simulink model "Model_AC_TES_Double_Coil"  (R2025b)
settings: Solver=VariableStepAuto  StartTime=0.0  StopTime=3600*9  RelTol=1e-3
model workspace (MAT data in the model file):
  COP = 3.9
  Delayfan = [30 1]
  P1 = 1.05
  P2 = 1.91
  P3 = 1.91
  P4 = 1.05
  Q_Cond = 4.361
  Q_Evap = 3.471
  T1 = 12
  T2 = 37.72
  T3 = 29.61
  T4 = 7.9
  T_Enviroment_C = 27.5
  T_Room_int_C = 28.6
  T_Tank_int_c = 30
  Wall_h_in = 12
  Wall_h_out = 38
  h1 = 522.3
  h2 = 528.6
  h3 = 253.4
  h4 = 253.4
  m_dot = 0.014
libraries: fl_lib x102, nesl_utility x62, SimscapeFluids_lib x31
(part 2 of 3)

== system Model_AC_TES_Double_Coil/22-12-2025 ==
  Clock2 : Clock
  Clock3 : Clock
  Constant1 : Constant
  Constant2 : Constant  Value=0
  Constant3 : Constant  Value=0
  Switch2 : Switch  Criteria=u2 > Threshold  Threshold=3600*10  SaturateOnIntegerOverflow=off  InputSameDT=off
  Switch3 : Switch  Criteria=u2 > Threshold  Threshold=3600*17  SaturateOnIntegerOverflow=off  InputSameDT=off
  Out1 : Outport
  wires:
  Constant3/1 -> Switch2/3
  Constant1/1 -> Switch2/1
  Clock2/1 -> Switch2/2
  Switch3/1 -> Out1/1
  Constant2/1 -> Switch3/1
  Clock3/1 -> Switch3/2
  Switch2/1 -> Switch3/3

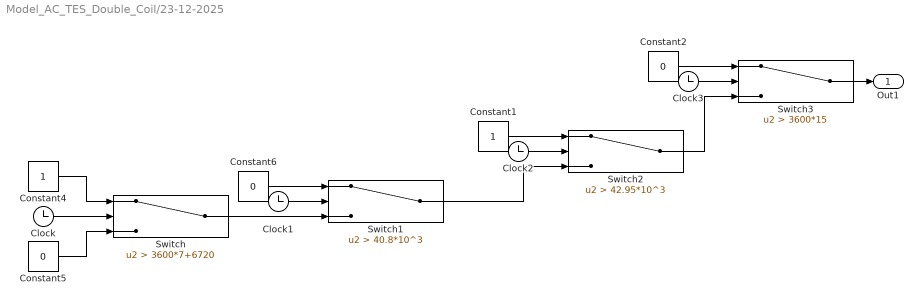
== system Model_AC_TES_Double_Coil/23-12-2025 ==
  Clock{,1..3} (4 alike) : Clock
  Constant1 : Constant
  Constant2 : Constant  Value=0
  Constant4 : Constant
  Constant5 : Constant  Value=0
  Constant6 : Constant  Value=0
  Switch : Switch  Criteria=u2 > Threshold  Threshold=3600*7+6720  SaturateOnIntegerOverflow=off  InputSameDT=off
  Switch1 : Switch  Criteria=u2 > Threshold  Threshold=40.8*10^3  SaturateOnIntegerOverflow=off  InputSameDT=off
  Switch2 : Switch  Criteria=u2 > Threshold  Threshold=42.95*10^3  SaturateOnIntegerOverflow=off  InputSameDT=off
  Switch3 : Switch  Criteria=u2 > Threshold  Threshold=3600*15  SaturateOnIntegerOverflow=off  InputSameDT=off
  Out1 : Outport
  wires:
  Constant6/1 -> Switch1/1
  Clock1/1 -> Switch1/2
  Switch/1 -> Switch1/3
  Constant4/1 -> Switch/1
  Clock/1 -> Switch/2
  Switch1/1 -> Switch2/3
  Constant5/1 -> Switch/3
  Constant1/1 -> Switch2/1
  Clock2/1 -> Switch2/2
  Switch3/1 -> Out1/1
  Constant2/1 -> Switch3/1
  Clock3/1 -> Switch3/2
  Switch2/1 -> Switch3/3

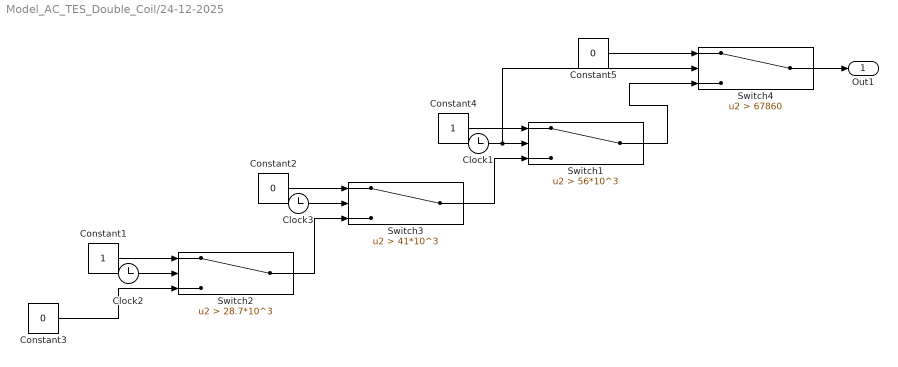
== system Model_AC_TES_Double_Coil/24-12-2025 ==
  Clock1 : Clock
  Clock2 : Clock
  Clock3 : Clock
  Constant1 : Constant
  Constant2 : Constant  Value=0
  Constant3 : Constant  Value=0
  Constant4 : Constant
  Constant5 : Constant  Value=0
  Switch1 : Switch  Criteria=u2 > Threshold  Threshold=56*10^3  SaturateOnIntegerOverflow=off  InputSameDT=off
  Switch2 : Switch  Criteria=u2 > Threshold  Threshold=28.7*10^3  SaturateOnIntegerOverflow=off  InputSameDT=off
  Switch3 : Switch  Criteria=u2 > Threshold  Threshold=41*10^3  SaturateOnIntegerOverflow=off  InputSameDT=off
  Switch4 : Switch  Criteria=u2 > Threshold  Threshold=67860  SaturateOnIntegerOverflow=off  InputSameDT=off
  Out1 : Outport
  wires:
  Constant3/1 -> Switch2/3
  Constant1/1 -> Switch2/1
  Clock2/1 -> Switch2/2
  Constant2/1 -> Switch3/1
  Clock3/1 -> Switch3/2
  Switch2/1 -> Switch3/3
  Switch1/1 -> Switch4/3
  Constant4/1 -> Switch1/1
  Clock1/1 -> Switch4/2, Switch1/2
  Switch3/1 -> Switch1/3
  Constant5/1 -> Switch4/1
  Switch4/1 -> Out1/1

== system Model_AC_TES_Double_Coil/25-12-2025 ==
  Clock1 : Clock
  Constant1 : Constant  Value=0
  Constant4 : Constant
  Constant5 : Constant  Value=0
  Switch1 : Switch  Criteria=u2 > Threshold  Threshold=28500  SaturateOnIntegerOverflow=off  InputSameDT=off
  Switch4 : Switch  Criteria=u2 > Threshold  Threshold=41600  SaturateOnIntegerOverflow=off  InputSameDT=off
  Out1 : Outport
  wires:
  Switch1/1 -> Switch4/3
  Constant4/1 -> Switch1/1
  Clock1/1 -> Switch4/2, Switch1/2
  Constant1/1 -> Switch1/3
  Constant5/1 -> Switch4/1
  Switch4/1 -> Out1/1

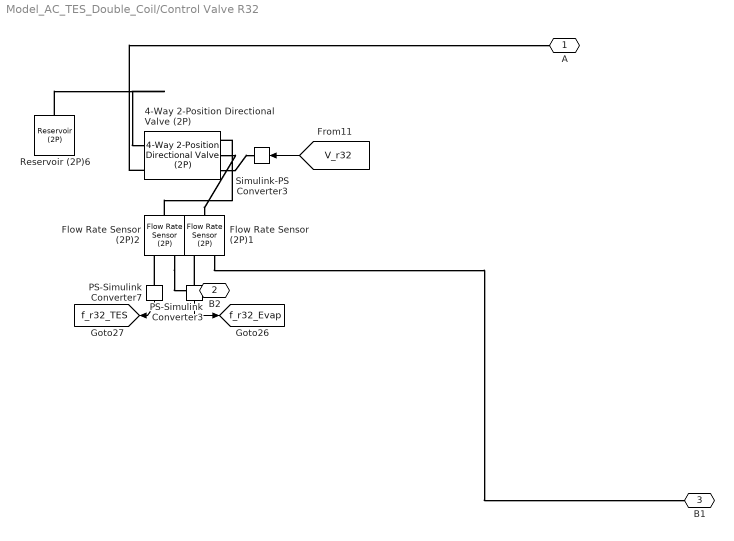
== system Model_AC_TES_Double_Coil/Control Valve R32 ==
  4-Way 2-Position Directional Valve (2P) : SimscapeFluids_lib/Two-Phase Fluid/Valves & Orifices/Directional Control Valves/4-Way 2-Position Directional Valve (2P)  open_orifices_pos=fluids.two_phase_fluid.valves_orifices.directional_control_valves.enum.OpenOrifices4Way2Position.PA  open_orifices_neg=fluids.two_phase_fluid.valves_orifices.directional_control_valves.enum.OpenOrifices4Way2Position.PB  area_spec=fluids.two_phase_fluid.valves_orifices.directional_control_valves.enum.AreaSpec.Identical  liquid_valve_parameterization=fluids.two_phase_fluid.valves_orifices.directional_control_valves.enum.LiquidOrificeParameterization.LinearArea  del_S_max=0.005 m  mdot_nominal_max=0.1 kg/s  delta_p_nominal_max=0.001 MPa  energy_spec=foundation.enum.energy_spec.temperature  p_inlet=0.101325 MPa  T_inlet=293.15 K  x_inlet=0  alpha_inlet=0  h_inlet=400 kJ/kg  u_inlet=400 kJ/kg  valve_area_max=1e-4 m^2  del_S_TLU=[0, .00125, .0025, .00375, .005] m  valve_area_TLU=[1e-10, 1e-05, 4e-05, 6e-05, .0001] m^2  Cd=0.64  pressure_recovery=false  leakage_fraction=1e-6  smoothing_factor=0.01  B_lam=0.999  tau_x=0.1 s  area=0.01 m^2  S_max_PA=0.01 m  del_S_max_PA=0.005 m  mdot_nominal_max_PA=0.1 kg/s  delta_p_nominal_max_PA=0.001 MPa  energy_spec_PA=foundation.enum.energy_spec.temperature  p_inlet_PA=0.101325 MPa  T_inlet_PA=293.15 K  x_inlet_PA=0  alpha_inlet_PA=0  h_inlet_PA=400 kJ/kg  u_inlet_PA=400 kJ/kg  valve_area_max_PA=1e-4 m^2  del_S_TLU_PA=[0, .00125, .0025, .00375, .005] m  valve_area_TLU_PA=[1e-10, 1e-05, 4e-05, 6e-05, .0001] m^2  mdot_nominal_const_PA=0.1 kg/s  delta_p_nominal_const_PA=0.001 MPa  valve_area_const_PA=1e-4 m^2  S_max_PB=0.01 m  del_S_max_PB=0.005 m  mdot_nominal_max_PB=0.1 kg/s  delta_p_nominal_max_PB=0.001 MPa  energy_spec_PB=foundation.enum.energy_spec.temperature  p_inlet_PB=0.101325 MPa  T_inlet_PB=293.15 K  x_inlet_PB=0  alpha_inlet_PB=0  h_inlet_PB=400 kJ/kg  u_inlet_PB=400 kJ/kg  valve_area_max_PB=1e-4 m^2  del_S_TLU_PB=[0, .00125, .0025, .00375, .005] m  valve_area_TLU_PB=[1e-10, 1e-05, 4e-05, 6e-05, .0001] m^2  mdot_nominal_const_PB=0.1 kg/s  delta_p_nominal_const_PB=0.001 MPa  valve_area_const_PB=1e-4 m^2  S_max_AT=-5e-3 m  del_S_max_AT=0.005 m  mdot_nominal_max_AT=0.1 kg/s  delta_p_nominal_max_AT=0.001 MPa  energy_spec_AT=foundation.enum.energy_spec.temperature  p_inlet_AT=0.101325 MPa  T_inlet_AT=293.15 K  x_inlet_AT=0  alpha_inlet_AT=0  h_inlet_AT=400 kJ/kg  u_inlet_AT=400 kJ/kg  valve_area_max_AT=1e-4 m^2  del_S_TLU_AT=[0, .00125, .0025, .00375, .005] m  valve_area_TLU_AT=[1e-10, 1e-05, 4e-05, 6e-05, .0001] m^2  mdot_nominal_const_AT=0.1 kg/s  delta_p_nominal_const_AT=0.001 MPa  valve_area_const_AT=1e-4 m^2  S_max_BT=5e-3 m  del_S_max_BT=0.005 m  mdot_nominal_max_BT=0.1 kg/s  delta_p_nominal_max_BT=0.001 MPa  energy_spec_BT=foundation.enum.energy_spec.temperature  p_inlet_BT=0.101325 MPa  T_inlet_BT=293.15 K  x_inlet_BT=0  alpha_inlet_BT=0  h_inlet_BT=400 kJ/kg  u_inlet_BT=400 kJ/kg  valve_area_max_BT=1e-4 m^2  del_S_TLU_BT=[0, .00125, .0025, .00375, .005] m  valve_area_TLU_BT=[1e-10, 1e-05, 4e-05, 6e-05, .0001] m^2  mdot_nominal_const_BT=0.1 kg/s  delta_p_nominal_const_BT=0.001 MPa  valve_area_const_BT=1e-4 m^2  vapor_valve_parameterization=fluids.two_phase_fluid.valves_orifices.enum.VaporOrificeParameterization.Cv  opening_characteristic=fluids.two_phase_fluid.valves_orifices.enum.OpeningCharacteristics.Linear  Cv_max=4  del_S_Cv_TLU=[0, .001, .002, .003, .004, .005] m  Cv_TLU=[1e-06, .8, 1.6, 2.4, 3.2, 4]  xT_Cv=0.7  Kv_max=3.6  del_S_Kv_TLU=[0, .001, .002, .003, .004, .005] m  Kv_TLU=[1e-06, .72, 1.44, 2.16, 2.88, 3.6]  xT_Kv=0.7  orifice_area_max=1e-4 m^2  del_S_orifice_area_TLU=[0, .001, .002, .003, .004, .005] m  orifice_area_TLU=[1e-10, 2e-05, 4e-05, 6e-05, 8e-05, .0001] m^2  Cv_const_PA=4  Cv_max_PA=4  del_S_Cv_TLU_PA=[0, .001, .002, .003, .004, .005] m  Cv_TLU_PA=[1e-06, .8, 1.6, 2.4, 3.2, 4]  xT_Cv_PA=0.7  Kv_const_PA=3.6  Kv_max_PA=3.6  del_S_Kv_TLU_PA=[0, .001, .002, .003, .004, .005] m  Kv_TLU_PA=[1e-06, .72, 1.44, 2.16, 2.88, 3.6]  xT_Kv_PA=0.7  orifice_area_const_PA=1e-4 m^2  orifice_area_max_PA=1e-4 m^2  del_S_orifice_area_TLU_PA=[0, .001, .002, .003, .004, .005] m  orifice_area_TLU_PA=[1e-10, 2e-05, 4e-05, 6e-05, 8e-05, .0001] m^2  Cv_const_PB=4  Cv_max_PB=4  del_S_Cv_TLU_PB=[0, .001, .002, .003, .004, .005] m  Cv_TLU_PB=[1e-06, .8, 1.6, 2.4, 3.2, 4]  xT_Cv_PB=0.7  Kv_const_PB=3.6  Kv_max_PB=3.6  del_S_Kv_TLU_PB=[0, .001, .002, .003, .004, .005] m  Kv_TLU_PB=[1e-06, .72, 1.44, 2.16, 2.88, 3.6]  xT_Kv_PB=0.7  orifice_area_const_PB=1e-4 m^2  orifice_area_max_PB=1e-4 m^2  del_S_orifice_area_TLU_PB=[0, .001, .002, .003, .004, .005] m  orifice_area_TLU_PB=[1e-10, 2e-05, 4e-05, 6e-05, 8e-05, .0001] m^2  Cv_const_AT=4  Cv_max_AT=4  del_S_Cv_TLU_AT=[0, .001, .002, .003, .004, .005] m  Cv_TLU_AT=[1e-06, .8, 1.6, 2.4, 3.2, 4]  xT_Cv_AT=0.7  Kv_const_AT=3.6  Kv_max_AT=3.6  del_S_Kv_TLU_AT=[0, .001, .002, .003, .004, .005] m  Kv_TLU_AT=[1e-06, .72, 1.44, 2.16, 2.88, 3.6]  xT_Kv_AT=0.7  orifice_area_const_AT=1e-4 m^2  orifice_area_max_AT=1e-4 m^2  del_S_orifice_area_TLU_AT=[0, .001, .002, .003, .004, .005] m  orifice_area_TLU_AT=[1e-10, 2e-05, 4e-05, 6e-05, 8e-05, .0001] m^2  Cv_const_BT=4  Cv_max_BT=4  del_S_Cv_TLU_BT=[0, .001, .002, .003, .004, .005] m  Cv_TLU_BT=[1e-06, .8, 1.6, 2.4, 3.2, 4]  xT_Cv_BT=0.7  Kv_const_BT=3.6  Kv_max_BT=3.6  del_S_Kv_TLU_BT=[0, .001, .002, .003, .004, .005] m  Kv_TLU_BT=[1e-06, .72, 1.44, 2.16, 2.88, 3.6]  xT_Kv_BT=0.7  orifice_area_const_BT=1e-4 m^2  orifice_area_max_BT=1e-4 m^2  del_S_orifice_area_TLU_BT=[0, .001, .002, .003, .004, .005] m  orifice_area_TLU_BT=[1e-10, 2e-05, 4e-05, 6e-05, 8e-05, .0001] m^2
      settings: InternalSimscapePortConfiguration="{\"Bottom\":[{\"id\":\"P\",\"label\":\"P\",\"type\":\"foundation.two_phase_fluid.two_phase_fluid\"},{\"id\":\"T\",\"label\":\"T\",\"type\":\"foundation.two_phase_fluid.two_phase_fluid\"}],\"Left\":[{\"id\":\"S\",\"label\":\"S\",\"type\":\"input\"}],\"Right\":[],\"Top\":[{\"id\":\"A\",\"label\":\"A\",\"type\":\"foundation.two_phase_fluid.two_phase_fluid\"},{\"id\":\"B\",\"label\":\"B\",\"type\":\"foundation.two_phase_fluid.two_phase_fluid\"}]}"
  Flow Rate Sensor (2P)1 : fl_lib/Two-Phase Fluid/Sensors/Flow Rate Sensor (2P)  mass_flow_measure=true  volumetric_flow_measure=false  energy_flow_measure=false
      settings: InternalSimscapePortConfiguration="{\"Bottom\":[],\"Left\":[{\"id\":\"A\",\"label\":\"A\",\"type\":\"foundation.two_phase_fluid.two_phase_fluid\"}],\"Right\":[{\"id\":\"B\",\"label\":\"B\",\"type\":\"foundation.two_phase_fluid.two_phase_fluid\"},{\"id\":\"M\",\"label\":\"M\",\"type\":\"output\"}],\"Top\":[]}"
  Flow Rate Sensor (2P)2 : fl_lib/Two-Phase Fluid/Sensors/Flow Rate Sensor (2P)  mass_flow_measure=true  volumetric_flow_measure=false  energy_flow_measure=false
      settings: InternalSimscapePortConfiguration="{\"Bottom\":[],\"Left\":[{\"id\":\"A\",\"label\":\"A\",\"type\":\"foundation.two_phase_fluid.two_phase_fluid\"}],\"Right\":[{\"id\":\"B\",\"label\":\"B\",\"type\":\"foundation.two_phase_fluid.two_phase_fluid\"},{\"id\":\"M\",\"label\":\"M\",\"type\":\"output\"}],\"Top\":[]}"
  PS-Simulink Converter3 : nesl_utility/PS-Simulink Converter  PhysicalDomain=network_engine_domain  SubClassName=ps_output  LeftPortType=input  RightPortType=output  PseudoPeriodic=off  Frequencies=[]  VectorFormat=inherit  Unit=inherit  AffineConversion=off
  PS-Simulink Converter7 : nesl_utility/PS-Simulink Converter  PhysicalDomain=network_engine_domain  SubClassName=ps_output  LeftPortType=input  RightPortType=output  PseudoPeriodic=off  Frequencies=[]  VectorFormat=inherit  Unit=inherit  AffineConversion=off
  Reservoir (2P)6 : fl_lib/Two-Phase Fluid/Elements/Reservoir (2P)  pressure_spec=foundation.enum.ReservoirPressureSpec2P.Specified  reservoir_pressure=0.8 MPa  reservoir_condensing_temperature=373.15 K  reservoir_evaporating_temperature=373.15 K  energy_spec=foundation.enum.ReservoirEnergySpec2P.Temperature  reservoir_temperature=8 degC  reservoir_quality=0.5  reservoir_void_fraction=0.5  reservoir_enthalpy=1500 kJ/kg  reservoir_internal_energy=1500 kJ/kg  reservoir_subcooling=5 deltaK  reservoir_superheating=5 deltaK  area_A=0.01 m^2
  Simulink-PS Converter3 : nesl_utility/Simulink-PS Converter  PhysicalDomain=network_engine_domain  SubClassName=ps_input  LeftPortType=input  RightPortType=output  PseudoPeriodic=off  Frequencies=[]  NoiseDistribution=none  NoiseParameters=[]  Unit=1  AffineConversion=off  FilteringAndDerivatives=provide  SimscapeFilterOrder=1  InputFilterTimeConstant=0.001  UdotUserProvided=0
  A : PMIOPort  Side=Left
  B2 : PMIOPort  Port=2  Side=Right
  B1 : PMIOPort  Port=3  Side=Right
  tag scope: f_r32_Evap=global, f_r32_TES=global
  wires:
  PS-Simulink Converter3/1 -> [f_r32_Evap]
  PS-Simulink Converter7/1 -> [f_r32_TES]
  [V_r32] -> Simulink-PS Converter3/1
  connections:
  4-Way 2-Position Directional Valve (2P)/LConn1 -- Simulink-PS Converter3/RConn1
  4-Way 2-Position Directional Valve (2P)/LConn2 -- Flow Rate Sensor (2P)1/LConn1
  PS-Simulink Converter7/LConn1 -- Flow Rate Sensor (2P)2/RConn2
  PS-Simulink Converter3/LConn1 -- Flow Rate Sensor (2P)1/RConn2
  Flow Rate Sensor (2P)2/LConn1 -- 4-Way 2-Position Directional Valve (2P)/LConn3
  Flow Rate Sensor (2P)2/RConn1 -- B2/RConn1
  4-Way 2-Position Directional Valve (2P)/RConn1 -- A/RConn1
  Flow Rate Sensor (2P)1/RConn1 -- B1/RConn1
  Reservoir (2P)6/LConn1 -- 4-Way 2-Position Directional Valve (2P)/RConn2

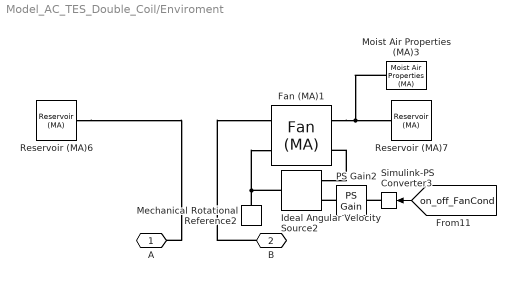
== system Model_AC_TES_Double_Coil/Enviroment ==
  Fan (MA)1 : SimscapeFluids_lib/Moist Air/Turbomachinery/Fan (MA)  fan_parameterization=fluids.moist_air.turbomachinery.enum.FanParameterization.Nominal  mechanical_power_spec=fluids.moist_air.turbomachinery.enum.FanMechanicalPowerSpec.Efficiency  flow_rate_nominal=4.5+0.2 m^3/s  pressure_nominal=5400 Pa  eta_nominal=0.40  power_nominal=1620 W  pressure_max=6400 Pa  flow_rate_max=4.5+0.3 m^3/s  omega_ref_nominal=1700 rpm  flow_rate_1D_TLU=[.0278, .0556, .0833, .111, .139, .167] m^3/s  pressure_1D_TLU=[6410, 6375, 6018, 5366, 4501, 3609] Pa  eta_1D_TLU=[.257, .394, .453, .47, .459, .415]  power_1D_TLU=[693, 900, 1107, 1267, 1363, 1452] W  omega_ref_1D=3000 rpm  rho_ref_1D=1.2 kg/m^3  omega_threshold_factor=1e-2  omega_dp_TLU=[2400; 3000; 3600] rpm  flow_rate_dp_TLU=[.0278, .0556, .0833, .111, .139, .167] m^3/s  pressure_dp_TLU=[4111, 4010, 3551, 2881, 2167, 1453; 6410, 6375, 6018, 5366, 4501, 3609; 9217, 9285, 9022, 8428, 7552, 6482] Pa  eta_dp_TLU=[.3, .434, .468, .459, .4, .3; .257, .394, .453, .47, .459, .415; .225, .359, .434, .461, .47, .459]  power_dp_TLU=[381, 514, 632, 697, 753, 809; 693, 900, 1107, 1267, 1363, 1452; 1139, 1438, 1732, 2029, 2233, 2358] W  rho_ref_dp=1.2 kg/m^3  omega_q_TLU=[2990; 3450; 3867] rpm  pressure_q_TLU=[31, 62, 93, 124] Pa  flow_rate_q_TLU=[.802, .759, .703, .611; .936, .902, .862, .81; 1.056, 1.027, .994, .956] m^3/s  eta_q_TLU=[.088, .162, .22, .261; .068, .128, .18, .222; .055, .105, .148, .188]  power_q_TLU=[283, 290, 297, 290; 427, 437, 445, 452; 595, 606, 625, 631] W  rho_ref_q=1.2 kg/m^3  diameter_ratio=1  mech_orientation=fluids.moist_air.turbomachinery.enum.FanMechanicalOrientation.Positive  area_A=0.01 m^2  area_B=0.01 m^2
      settings: InternalSimscapePortConfiguration="{\"Bottom\":[],\"Left\":[{\"id\":\"A\",\"label\":\"A\",\"type\":\"foundation.moist_air.moist_air\"},{\"id\":\"C\",\"label\":\"C\",\"type\":\"foundation.mechanical.rotational.rotational\"}],\"Right\":[{\"id\":\"B\",\"label\":\"B\",\"type\":\"foundation.moist_air.moist_air\"},{\"id\":\"R\",\"label\":\"R\",\"type\":\"foundation.mechanical.rotational.rotational\"}],\"Top\":[]}"
  Ideal Angular Velocity Source2 : fl_lib/Mechanical/Mechanical Sources/Ideal Angular Velocity Source
  Mechanical Rotational Reference2 : fl_lib/Mechanical/Rotational Elements/Mechanical Rotational Reference
  Moist Air Properties (MA)3 : fl_lib/Moist Air/Utilities/Moist Air Properties (MA)  R_a=287.047 J/(K*kg)  T_TLU=[-56.55, -50 : 10 : -10, -5 : 1 : 5, 10 : 10 : 350]' degC  h_a_TLU=[342.414066793634; 349.003411914139; 359.061417476782; 369.117728274935; 379.173188407993; 389.228602960013; 394.256538873206; 395.262156814682; 396.26778682262; 397.27342967397; 398.279086145689; 399.284757014822; 400.290443058569; 401.296145054364; 402.301863779931; 403.307600013352; 404.313354533128; 409.342428711098; 419.402397945314; 429.465451846544; 439.532387826623; 449.604014793745; 459.68115297076; 469.764632657687; 479.855292205971; 489.953975419749; 500.06152856014; 510.178797098051; 520.306622336267; 530.445838000969; 540.597266885076; 550.761717610289; 560.939981561004; 571.132830031086; 581.341011613777; 591.565249855533; 601.806241186423; 612.064653132654; 622.341122810862; 632.636255698901; 642.95062467384; 653.284769304793; 663.639195385783; 674.014374692179; 684.410744943084; 694.828709951456; 705.268639943519; 715.730872029167; 726.215710805484; 736.723429076127; 747.254268670154; 757.808441344776] kJ/kg  mu_a_TLU=[14.2568884161326; 14.6140128551699; 15.151727785151; 15.6806860927178; 16.201235181264; 16.7137043838401; 16.9670072430524; 17.017438132541; 17.0677931537044; 17.1180726001803; 17.1682767640582; 17.2184059358881; 17.2684604046898; 17.318440457962; 17.3683463816913; 17.4181784603614; 17.467936976962; 17.7156359301048; 18.2056752419787; 18.6887904184394; 19.1652345249932; 19.6352479488881; 20.099059157425; 20.5568854116507; 21.008933436444; 21.4554000485251; 21.8964727442509; 22.3323302492491; 22.7631430320408; 23.1890737838183; 23.6102778665211; 24.0269037312887; 24.4390933092858; 24.8469823767971; 25.2507008963847; 25.6503733357905; 26.0461189661617; 26.438052141067; 26.8262825576728; 27.210915501349; 27.5920520748824; 27.969789413389; 28.3442208859359; 28.7154362848061; 29.0835220032714; 29.4485612026716; 29.8106339695395; 30.169817463453; 30.5261860562487; 30.8798114631771; 31.2307628665438; 31.5791070323335] s*uPa  k_a_TLU=[19.8808491891482; 20.4162457047568; 21.2248745869044; 22.0232455041378; 22.8117316528767; 23.59069155438; 23.9767077285082; 24.0536401764626; 24.130482853517; 24.2072360894785; 24.2839002127411; 24.3604755502875; 24.4369624276914; 24.5133611691197; 24.5896720973349; 24.6658955336975; 24.7420317981691; 25.1214166432482; 25.8738284673185; 26.6180151791963; 27.3542675863918; 28.0828636150405; 28.8040688184917; 29.5181369069754; 30.2253102842368; 30.9258205811167; 31.6198891790667; 32.307727718801; 32.989538590917; 33.6655154065126; 34.3358434467079; 35.0007000906151; 35.6602552217624; 36.314671613305; 36.9641052925838; 37.6087058857479; 38.2486169432557; 38.8839762471259; 39.5149161008418; 40.1415636028127; 40.7640409042923; 41.3824654526272; 41.9969502206863; 42.6076039232795; 43.2145312213471; 43.8178329146528; 44.4176061236819; 45.0139444614019; 45.6069381955058; 46.1966744017242; 46.7832371087507; 47.3667074352967] mW/(K*m)  p_min=1 kPa  p_max=inf MPa  T_min=-56.55 degC  T_max=350 degC  properties_range_check=simscape.enum.assert.action.error  p_atm=0.101325 MPa  T_atm=20 degC  enable_droplets=false  R_w=461.523 J/(K*kg)  p_ws_TLU=[1.71168953425982e-06; 3.93770601979424e-06; 1.28411717710344e-05; 3.80051394873809e-05; .00010323902900209; .000259873810798063; .000401741022116384; .000437454836117844; .000476040820618202; .000517704666185737; .000562664883741207; .000611212677444345; .000657085634113763; .000705985593917791; .00075808051438111; .000813548355379396; .000872575113841924; .00122819910164487; .00233931836947519; .00424697076171126; .00738493802968097; .012351945812707; .0199464343236764; .0312009300307261; .0474144740241604; .0701817658485933; .101417996663294; .143378712947169; .198674420476403; .270279976781692; .361539099388177; .476164537971214; .618234621423587; .792187006980199; 1.00281053608169; 1.25523615516845; 1.55492790046272; 1.90767499353199; 2.31958617020155; 2.79708749692822; 3.34692514426746; 3.97617493064794; 4.69226099229504; 5.50298678300951; 6.41658290952841; 7.44177834442093; 8.58790494083256; 9.86505121117553; 11.284292927457; 12.8580516000122; 14.6006773719404; 16.5294151389953] MPa  h_w_vap_TLU=[2836.88241275372; 2837.81392500514; 2838.63937175807; 2838.7309929628; 2838.06905313927; 2836.62597341095; 2835.60023952573; 2835.37006381376; 2835.13143158077; 2834.88429145066; 2834.62859062897; 2500.93420564316; 2498.55452890293; 2496.17317793437; 2493.7941260618; 2491.41713708944; 2489.04199020767; 2477.18706302224; 2453.51925941961; 2429.81122987564; 2405.97728678685; 2381.94712654051; 2357.65452030374; 2333.03120800924; 2308.00352809267; 2282.49062771796; 2256.40372152657; 2229.64615315163; 2202.11407337172; 2173.6974807639; 2144.28128268553; 2113.74600964951; 2081.9678834089; 2048.81807129851; 2014.16109962579; 1977.85249331179; 1939.73572816654; 1899.63852389863; 1857.36838273035; 1812.70710332357; 1765.4037880462; 1715.16561416478; 1661.64526339623; 1604.4232249434; 1542.98206457018; 1476.66790089115; 1404.63083498414; 1325.72875296442; 1238.36212284382; 1140.16281350074; 1027.31658328826; 892.746804215825] kJ/kg  h_w_TLU=[2396.53078650168; 2408.65722023252; 2427.16766028467; 2445.66624034104; 2464.1379798878; 2482.5594701893; 2491.7412703989; 2493.57467660537; 2495.40699233755; 2497.23816944599; 2499.06815833272; 2500.89261781717; 2502.73123919979; 2504.56496564907; 2506.39800457704; 2508.23033644628; 2510.06194120626; 2519.20831890725; 2537.43340437276; 2555.54520329515; 2573.51032237465; 2591.28888786817; 2608.83487221908; 2626.09640083333; 2643.01588134754; 2659.53001419864; 2675.5827869577; 2696.18462565746; 2716.49989554204; 2736.6235211014; 2756.61216047677; 2776.50561774616; 2796.33378923373; 2816.11979584021; 2835.88181424959; 2855.6343057571; 2875.38889328914; 2895.15500578618; 2914.94035966265; 2934.75132291939; 2954.59319332093; 2974.47041287496; 2994.38673461102; 3014.34535330297; 3034.34900869544; 3054.40006758361; 3074.50058949656; 3094.65237956705; 3114.85703131193; 3135.11596141057; 3155.43043809331; 3175.80160439414] kJ/kg  mu_w_TLU=[6.9886414857741; 7.21462000349698; 7.55962537406626; 7.90463074463554; 8.24963611520482; 8.5946414857741; 8.76714417105874; 8.80164470811567; 8.8361452451726; 8.87064578222952; 8.90514631928645; 8.93964685634338; 8.97414739340031; 9.00294911497154; 9.0318980288863; 9.06099135942002; 9.09022638806001; 9.23843559844524; 9.5440595677542; 9.86015858692705; 10.1848429274122; 10.5164578096049; 10.8535319382781; 11.1947482575333; 11.5389294976352; 11.8850331780701; 12.2322493177351; 12.6188533568459; 13.0082793358938; 13.4003380262893; 13.7948421428098; 14.1916095618232; 14.590464747099; 14.9912394314964; 15.3937729006119; 15.7979120385447; 16.203511226482; 16.610432150303; 17.0185435533718; 17.4277209582061; 17.8378463726577; 18.2488079909412; 18.6604998963166; 19.0728217698535; 19.485678608085; 19.8989804512625; 20.3126421231677; 20.7265829829225; 21.1407266888906; 21.5550009745266; 21.969337435876; 22.3836713303269] s*uPa  k_w_TLU=[12.4916816538045; 12.9847788176262; 13.737598915064; 14.4904190125018; 15.2432391099396; 15.9960592073774; 16.3724692560963; 16.4477512658401; 16.5230332755839; 16.5983152853277; 16.6735972950715; 16.7488793048152; 16.824161314559; 16.8886088206517; 16.9532779906513; 17.0181691764255; 17.083282769915; 17.4122036181723; 18.0870861656185; 18.7855813517187; 19.5093466408385; 20.2607864040347; 21.0430876297671; 21.8602068151121; 22.7168164077153; 23.6182141540994; 24.5698636875305; 25.4024944426483; 26.2458938647479; 27.1009155051916; 27.968142896353; 28.8479507975112; 29.7405485790829; 30.646029672269; 31.5643932662527; 32.4955693285114; 33.4394360046859; 34.3958329885356; 35.3645718140131; 36.3454437886179; 37.3382261129791; 38.3426866012072; 39.3585873185985; 40.3856873794121; 41.4237450915028; 42.4725195920623; 43.5317720862424; 44.6012667755489; 45.6807715437344; 46.7700584531355; 47.8689040929333; 48.9770898119082] mW/(K*m)  D_w=25 mm^2/s  trace_gas_model=foundation.enum.trace_gas_model.none  R_g=188.923 J/(K*kg)  h_g_TLU=[439.555216276024; 444.670268214299; 452.538618857965; 460.487124266174; 468.522588773143; 476.64941595933; 480.747985385885; 481.570543185868; 482.394052396612; 483.218514286302; 484.043930026094; 484.87030069324; 485.697627274149; 486.525910667382; 487.355151686572; 488.185351063277; 489.016509449741; 493.186704132078; 501.599194941473; 510.107689945701; 518.711611059603; 527.410026767716; 536.20176474847; 545.085474167968; 554.059675464379; 563.122805439004; 572.273250917104; 581.509372969931; 590.829525041787; 600.232066635428; 609.715373504524; 619.277845094572; 628.91790983254; 638.634028741375; 648.424697754692; 658.288449028076; 668.22385148184; 678.229510761734; 688.30406876583; 698.446202855373; 708.654624842952; 718.928079831753; 729.265344963773; 739.665228122078; 750.126566621791; 760.648225916092; 771.229098336723; 781.86810188302; 792.564179069104; 803.316295835373; 814.123440527678; 824.984622945405] kJ/kg  mu_g_TLU=[10.9386626034033; 11.2618160869372; 11.7542862475187; 12.2454955799777; 12.7352208796158; 13.2232325321233; 13.4665248390743; 13.5151226761166; 13.5636997995993; 13.6122559954699; 13.6607910510226; 13.709304754931; 13.757796897279; 13.8062672695897; 13.8547156648526; 13.9031418775498; 13.9515457036801; 14.1932220047332; 14.6747828595747; 15.153802214283; 15.6301123398299; 16.1035631756244; 16.574022106427; 17.0413733976215; 17.5055174102327; 17.9663696812767; 18.4238599299346; 18.8779310322956; 19.3285379947687; 19.7756469471288; 20.2192341695255; 20.6592851629269; 21.0957937689132; 21.5287613421341; 21.9581959768344; 22.3841117874779; 22.8065282425078; 23.2254695495877; 23.6409640901974; 24.0530439011453; 24.4617442003854; 24.8671029544344; 25.269160484669; 25.6679591098169; 26.0635428220247; 26.4559569939835; 26.8452481147025; 27.2314635516519; 27.6146513371198; 27.9948599767665; 28.3721382784874; 28.74653519983] s*uPa  k_g_TLU=[10.7373095949238; 11.1772934980884; 11.862915506018; 12.5638333280734; 13.2785475592421; 14.005722199619; 14.3736017704762; 14.4475028211958; 14.5215096973787; 14.5956213250986; 14.6698366403414; 14.7441545888563; 14.8185741260114; 14.8930942166532; 14.9677138349692; 15.0424319643548; 15.1172475972825; 15.4927536712633; 16.2505237772467; 17.0165521650722; 17.7899991951805; 18.5700903932503; 19.3561099002839; 20.1473949639617; 20.9433312278214; 21.7433486448307; 22.5469178892132; 23.3535471729555; 24.1627793965491; 24.9741895799701; 25.7873825314493; 26.6019907190427; 27.4176723115859; 28.2341093347412; 29.0510055857402; 29.8680879651392; 30.6851034165693; 31.5018116707882; 32.3179924018673; 33.1334410491403; 33.9479677779769; 34.7613965127281; 35.5735640361829; 36.3843191504339; 37.1935218945334; 38.0010428147395; 38.80676228352; 39.6105698638057; 40.412363715274; 41.2120500397018; 42.0095425626597; 42.8047620490288] mW/(K*m)  D_g=16 mm^2/s
  PS Gain2 : fl_lib/Physical Signals/Functions/PS Gain  gain=1700 rpm
  Reservoir (MA)6 : fl_lib/Moist Air/Elements/Reservoir (MA)  pressure_input=false  pressure_spec=foundation.enum.pressure_spec.atmospheric  reservoir_pressure=0.101325 MPa  temperature_input=false  temperature_spec=foundation.enum.temperature_spec.specified  reservoir_temperature=273.15+T_Enviroment_C K  humidity_input=false  humidity_spec=foundation.enum.HumiditySpec.RelativeHumidity  reservoir_RH=0.5  reservoir_x_w=0.01  reservoir_y_w=0.01  reservoir_HR=0.01  reservoir_Tw=287 K  trace_gas_input=false  trace_gas_spec=foundation.enum.trace_gas_spec.mass_fraction  reservoir_x_g=0.001  reservoir_y_g=0.001  water_droplets_input=false  reservoir_r_d=0  RH_ws=1  area_A=0.01 m^2  input_error_spec=foundation.enum.input_range_error.warn
  Reservoir (MA)7 : fl_lib/Moist Air/Elements/Reservoir (MA)  pressure_input=false  pressure_spec=foundation.enum.pressure_spec.atmospheric  reservoir_pressure=0.101325 MPa  temperature_input=false  temperature_spec=foundation.enum.temperature_spec.specified  reservoir_temperature=T_Enviroment_C+273.15 K  humidity_input=false  humidity_spec=foundation.enum.HumiditySpec.RelativeHumidity  reservoir_RH=0.5  reservoir_x_w=0.01  reservoir_y_w=0.01  reservoir_HR=0.01  reservoir_Tw=287 K  trace_gas_input=false  trace_gas_spec=foundation.enum.trace_gas_spec.mass_fraction  reservoir_x_g=0.001  reservoir_y_g=0.001  water_droplets_input=false  reservoir_r_d=0  RH_ws=1  area_A=0.01 m^2  input_error_spec=foundation.enum.input_range_error.warn
  Simulink-PS Converter3 : nesl_utility/Simulink-PS Converter  PhysicalDomain=network_engine_domain  SubClassName=ps_input  LeftPortType=input  RightPortType=output  PseudoPeriodic=off  Frequencies=[]  NoiseDistribution=none  NoiseParameters=[]  Unit=1  AffineConversion=off  FilteringAndDerivatives=provide  SimscapeFilterOrder=1  InputFilterTimeConstant=0.001  UdotUserProvided=0
  A : PMIOPort  Side=Left
  B : PMIOPort  Port=2  Side=Right
  wires:
  [on_off_FanCond] -> Simulink-PS Converter3/1
  connections:
  Fan (MA)1/LConn1 -- Moist Air Properties (MA)3/RConn1 -- Reservoir (MA)7/LConn1
  Ideal Angular Velocity Source2/LConn1 -- Fan (MA)1/RConn2 -- Mechanical Rotational Reference2/LConn1
  PS Gain2/RConn1 -- Ideal Angular Velocity Source2/RConn1
  Simulink-PS Converter3/RConn1 -- PS Gain2/LConn1
  B/RConn1 -- Fan (MA)1/RConn1
  Ideal Angular Velocity Source2/RConn2 -- Fan (MA)1/LConn2
  Reservoir (MA)6/LConn1 -- A/RConn1

== system Model_AC_TES_Double_Coil/Fan Drive ==
  Ideal Angular Velocity Source1 : fl_lib/Mechanical/Mechanical Sources/Ideal Angular Velocity Source
  Mechanical Rotational Reference1 : fl_lib/Mechanical/Rotational Elements/Mechanical Rotational Reference
  PS Gain1 : fl_lib/Physical Signals/Functions/PS Gain  gain=1200 rpm
  Simulink-PS Converter : nesl_utility/Simulink-PS Converter  PhysicalDomain=network_engine_domain  SubClassName=ps_input  LeftPortType=input  RightPortType=output  PseudoPeriodic=off  Frequencies=[]  NoiseDistribution=none  NoiseParameters=[]  Unit=1  AffineConversion=off  FilteringAndDerivatives=provide  SimscapeFilterOrder=1  InputFilterTimeConstant=0.001  UdotUserProvided=0
  C : PMIOPort  Side=Right
  R : PMIOPort  Port=2  Side=Left
  wires:
  [on_off_FanEvap] -> Simulink-PS Converter/1
  connections:
  Ideal Angular Velocity Source1/RConn2 -- C/RConn1
  PS Gain1/RConn1 -- Ideal Angular Velocity Source1/RConn1
  Simulink-PS Converter/RConn1 -- PS Gain1/LConn1
  Ideal Angular Velocity Source1/LConn1 -- R/RConn1 -- Mechanical Rotational Reference1/LConn1

== system Model_AC_TES_Double_Coil/Flow rate sensor : R32 ==
  Display1 : Display
  Flow Rate Sensor (2P) : fl_lib/Two-Phase Fluid/Sensors/Flow Rate Sensor (2P)  mass_flow_measure=true  volumetric_flow_measure=false  energy_flow_measure=true
      settings: InternalSimscapePortConfiguration="{\"Bottom\":[{\"id\":\"PHI\",\"label\":\"φ\",\"type\":\"output\"}],\"Left\":[{\"id\":\"A\",\"label\":\"A\",\"type\":\"foundation.two_phase_fluid.two_phase_fluid\"}],\"Right\":[{\"id\":\"B\",\"label\":\"B\",\"type\":\"foundation.two_phase_fluid.two_phase_fluid\"},{\"id\":\"M\",\"label\":\"M\",\"type\":\"output\"}],\"Top\":[]}"
  PS-Simulink Converter2 : nesl_utility/PS-Simulink Converter  PhysicalDomain=network_engine_domain  SubClassName=ps_output  LeftPortType=input  RightPortType=output  PseudoPeriodic=off  Frequencies=[]  VectorFormat=inherit  Unit=inherit  AffineConversion=off
  B : PMIOPort  Side=Right
  A : PMIOPort  Port=2  Side=Left
  tag scope: f_r32_main=global
  wires:
  PS-Simulink Converter2/1 -> Display1/1, [f_r32_main]
  connections:
  Flow Rate Sensor (2P)/RConn2 -- PS-Simulink Converter2/LConn1
  A/RConn1 -- Flow Rate Sensor (2P)/LConn1
  Flow Rate Sensor (2P)/RConn1 -- B/RConn1

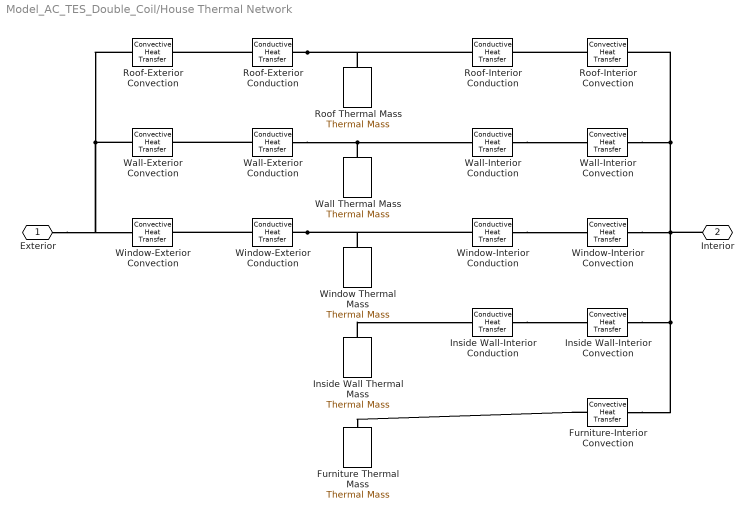
== system Model_AC_TES_Double_Coil/House Thermal Network ==
  Furniture Thermal Mass : fl_lib/Thermal/Thermal Elements/Thermal Mass  mass_type=foundation.enum.constant_variable.constant  mass=M_furniture kg  sp_heat=cp_furniture J/(K*kg)  mass_min=1e-6 kg  num_ports=foundation.enum.numPorts2.one  m_specify=off  m_priority=High  m=1 kg  m_nominal_specify=off  m_nominal_value=1  m_nominal_unit=kg  T_specify=on  T_priority=High  T=T_init_furniture degC  T_nominal_specify=off  T_nominal_value=1  T_nominal_unit=K  Q_specify=off  Q_priority=None  Q=0 W  Q_nominal_specify=off  Q_nominal_value=1  Q_nominal_unit=W
  Furniture-Interior Convection : fl_lib/Thermal/Thermal Elements/Convective Heat Transfer  thermal_type=foundation.enum.constant_variable.constant  area=area_furniture m^2  heat_tr_coeff=hc_furniture_interior W/(K*m^2)  min_heat_tr_coeff=1e-3 W/(K*m^2)  T_specify=off  T_priority=None  T=0 K  T_nominal_specify=off  T_nominal_value=1  T_nominal_unit=K  Q_specify=off  Q_priority=None  Q=0 W  Q_nominal_specify=off  Q_nominal_value=1  Q_nominal_unit=W
  Inside Wall Thermal Mass : fl_lib/Thermal/Thermal Elements/Thermal Mass  mass_type=foundation.enum.constant_variable.constant  mass=rho_wall_inside * area_wall_inside * thickness_wall_inside kg  sp_heat=cp_wall_inside J/(K*kg)  mass_min=1e-6 kg  num_ports=foundation.enum.numPorts2.one  m_specify=off  m_priority=High  m=1 kg  m_nominal_specify=off  m_nominal_value=1  m_nominal_unit=kg  T_specify=on  T_priority=High  T=T_init_wall_inside degC  T_nominal_specify=off  T_nominal_value=1  T_nominal_unit=K  Q_specify=off  Q_priority=None  Q=0 W  Q_nominal_specify=off  Q_nominal_value=1  Q_nominal_unit=W
  Inside Wall-Interior Conduction : fl_lib/Thermal/Thermal Elements/Conductive Heat Transfer  thermal_type=foundation.enum.ConstantVariableTabulated.Constant  wall_geometry=foundation.enum.ConductionWallGeometry.Planar  area=2 * area_wall_inside m^2  thickness=thickness_wall_inside / 2 m  d_in=0.05 m  d_out=0.1 m  L=1 m  th_cond_min=10 W/(K*m)  th_cond=k_wall_inside W/(K*m)  th_cond_TLU=[413, 401, 392, 383, 371, 357, 342] W/(K*m)  temp_TLU=[200, 273, 400, 600, 800, 1000, 1200] K  T_specify=off  T_priority=None  T=0 K  T_nominal_specify=off  T_nominal_value=1  T_nominal_unit=K  Q_specify=off  Q_priority=None  Q=0 W  Q_nominal_specify=off  Q_nominal_value=1  Q_nominal_unit=W
  Inside Wall-Interior Convection : fl_lib/Thermal/Thermal Elements/Convective Heat Transfer  thermal_type=foundation.enum.constant_variable.constant  area=2 * area_wall_inside m^2  heat_tr_coeff=hc_wall_inside_interior W/(K*m^2)  min_heat_tr_coeff=1e-3 W/(K*m^2)  T_specify=off  T_priority=None  T=0 K  T_nominal_specify=off  T_nominal_value=1  T_nominal_unit=K  Q_specify=off  Q_priority=None  Q=0 W  Q_nominal_specify=off  Q_nominal_value=1  Q_nominal_unit=W
  Roof Thermal Mass : fl_lib/Thermal/Thermal Elements/Thermal Mass  mass_type=foundation.enum.constant_variable.constant  mass=rho_roof * area_roof * thickness_roof kg  sp_heat=cp_roof J/(K*kg)  mass_min=1e-6 kg  num_ports=foundation.enum.numPorts2.one  m_specify=off  m_priority=High  m=1 kg  m_nominal_specify=off  m_nominal_value=1  m_nominal_unit=kg  T_specify=on  T_priority=High  T=T_init_roof degC  T_nominal_specify=off  T_nominal_value=1  T_nominal_unit=K  Q_specify=off  Q_priority=None  Q=0 W  Q_nominal_specify=off  Q_nominal_value=1  Q_nominal_unit=W
  Roof-Exterior Conduction : fl_lib/Thermal/Thermal Elements/Conductive Heat Transfer  thermal_type=foundation.enum.ConstantVariableTabulated.Constant  wall_geometry=foundation.enum.ConductionWallGeometry.Planar  area=area_roof m^2  thickness=thickness_roof / 2 m  d_in=0.05 m  d_out=0.1 m  L=1 m  th_cond_min=10 W/(K*m)  th_cond=k_roof W/(K*m)  th_cond_TLU=[413, 401, 392, 383, 371, 357, 342] W/(K*m)  temp_TLU=[200, 273, 400, 600, 800, 1000, 1200] K  T_specify=off  T_priority=None  T=0 K  T_nominal_specify=off  T_nominal_value=1  T_nominal_unit=K  Q_specify=off  Q_priority=None  Q=0 W  Q_nominal_specify=off  Q_nominal_value=1  Q_nominal_unit=W
  Roof-Exterior Convection : fl_lib/Thermal/Thermal Elements/Convective Heat Transfer  thermal_type=foundation.enum.constant_variable.constant  area=area_roof m^2  heat_tr_coeff=hc_roof_exterior W/(K*m^2)  min_heat_tr_coeff=1e-3 W/(K*m^2)  T_specify=off  T_priority=None  T=0 K  T_nominal_specify=off  T_nominal_value=1  T_nominal_unit=K  Q_specify=off  Q_priority=None  Q=0 W  Q_nominal_specify=off  Q_nominal_value=1  Q_nominal_unit=W
  Roof-Interior Conduction : fl_lib/Thermal/Thermal Elements/Conductive Heat Transfer  thermal_type=foundation.enum.ConstantVariableTabulated.Constant  wall_geometry=foundation.enum.ConductionWallGeometry.Planar  area=area_roof m^2  thickness=thickness_roof / 2 m  d_in=0.05 m  d_out=0.1 m  L=1 m  th_cond_min=10 W/(K*m)  th_cond=k_roof W/(K*m)  th_cond_TLU=[413, 401, 392, 383, 371, 357, 342] W/(K*m)  temp_TLU=[200, 273, 400, 600, 800, 1000, 1200] K  T_specify=off  T_priority=None  T=0 K  T_nominal_specify=off  T_nominal_value=1  T_nominal_unit=K  Q_specify=off  Q_priority=None  Q=0 W  Q_nominal_specify=off  Q_nominal_value=1  Q_nominal_unit=W
  Roof-Interior Convection : fl_lib/Thermal/Thermal Elements/Convective Heat Transfer  thermal_type=foundation.enum.constant_variable.constant  area=area_roof m^2  heat_tr_coeff=hc_roof_interior W/(K*m^2)  min_heat_tr_coeff=1e-3 W/(K*m^2)  T_specify=off  T_priority=None  T=0 K  T_nominal_specify=off  T_nominal_value=1  T_nominal_unit=K  Q_specify=off  Q_priority=None  Q=0 W  Q_nominal_specify=off  Q_nominal_value=1  Q_nominal_unit=W
  Wall Thermal Mass : fl_lib/Thermal/Thermal Elements/Thermal Mass  mass_type=foundation.enum.constant_variable.constant  mass=rho_wall * area_wall * thickness_wall kg  sp_heat=cp_wall J/(K*kg)  mass_min=1e-6 kg  num_ports=foundation.enum.numPorts2.one  m_specify=off  m_priority=High  m=1 kg  m_nominal_specify=off  m_nominal_value=1  m_nominal_unit=kg  T_specify=on  T_priority=High  T=T_init_wall degC  T_nominal_specify=off  T_nominal_value=1  T_nominal_unit=K  Q_specify=off  Q_priority=None  Q=0 W  Q_nominal_specify=off  Q_nominal_value=1  Q_nominal_unit=W
  Wall-Exterior Conduction : fl_lib/Thermal/Thermal Elements/Conductive Heat Transfer  thermal_type=foundation.enum.ConstantVariableTabulated.Constant  wall_geometry=foundation.enum.ConductionWallGeometry.Planar  area=area_wall m^2  thickness=thickness_wall / 2 m  d_in=0.05 m  d_out=0.1 m  L=1 m  th_cond_min=10 W/(K*m)  th_cond=k_wall W/(K*m)  th_cond_TLU=[413, 401, 392, 383, 371, 357, 342] W/(K*m)  temp_TLU=[200, 273, 400, 600, 800, 1000, 1200] K  T_specify=off  T_priority=None  T=0 K  T_nominal_specify=off  T_nominal_value=1  T_nominal_unit=K  Q_specify=off  Q_priority=None  Q=0 W  Q_nominal_specify=off  Q_nominal_value=1  Q_nominal_unit=W
  Wall-Exterior Convection : fl_lib/Thermal/Thermal Elements/Convective Heat Transfer  thermal_type=foundation.enum.constant_variable.constant  area=area_wall m^2  heat_tr_coeff=hc_wall_exterior W/(K*m^2)  min_heat_tr_coeff=1e-3 W/(K*m^2)  T_specify=off  T_priority=None  T=0 K  T_nominal_specify=off  T_nominal_value=1  T_nominal_unit=K  Q_specify=off  Q_priority=None  Q=0 W  Q_nominal_specify=off  Q_nominal_value=1  Q_nominal_unit=W
  Wall-Interior Conduction : fl_lib/Thermal/Thermal Elements/Conductive Heat Transfer  thermal_type=foundation.enum.ConstantVariableTabulated.Constant  wall_geometry=foundation.enum.ConductionWallGeometry.Planar  area=area_wall m^2  thickness=thickness_wall / 2 m  d_in=0.05 m  d_out=0.1 m  L=1 m  th_cond_min=10 W/(K*m)  th_cond=k_wall W/(K*m)  th_cond_TLU=[413, 401, 392, 383, 371, 357, 342] W/(K*m)  temp_TLU=[200, 273, 400, 600, 800, 1000, 1200] K  T_specify=off  T_priority=None  T=0 K  T_nominal_specify=off  T_nominal_value=1  T_nominal_unit=K  Q_specify=off  Q_priority=None  Q=0 W  Q_nominal_specify=off  Q_nominal_value=1  Q_nominal_unit=W
  Wall-Interior Convection : fl_lib/Thermal/Thermal Elements/Convective Heat Transfer  thermal_type=foundation.enum.constant_variable.constant  area=area_wall m^2  heat_tr_coeff=hc_wall_interior W/(K*m^2)  min_heat_tr_coeff=1e-3 W/(K*m^2)  T_specify=off  T_priority=None  T=0 K  T_nominal_specify=off  T_nominal_value=1  T_nominal_unit=K  Q_specify=off  Q_priority=None  Q=0 W  Q_nominal_specify=off  Q_nominal_value=1  Q_nominal_unit=W
  Window Thermal Mass : fl_lib/Thermal/Thermal Elements/Thermal Mass  mass_type=foundation.enum.constant_variable.constant  mass=rho_window * area_window * thickness_window kg  sp_heat=cp_window J/(K*kg)  mass_min=1e-6 kg  num_ports=foundation.enum.numPorts2.one  m_specify=off  m_priority=High  m=1 kg  m_nominal_specify=off  m_nominal_value=1  m_nominal_unit=kg  T_specify=on  T_priority=High  T=T_init_window degC  T_nominal_specify=off  T_nominal_value=1  T_nominal_unit=K  Q_specify=off  Q_priority=None  Q=0 W  Q_nominal_specify=off  Q_nominal_value=1  Q_nominal_unit=W
  Window-Exterior Conduction : fl_lib/Thermal/Thermal Elements/Conductive Heat Transfer  thermal_type=foundation.enum.ConstantVariableTabulated.Constant  wall_geometry=foundation.enum.ConductionWallGeometry.Planar  area=area_window m^2  thickness=thickness_window / 2 m  d_in=0.05 m  d_out=0.1 m  L=1 m  th_cond_min=10 W/(K*m)  th_cond=k_window W/(K*m)  th_cond_TLU=[413, 401, 392, 383, 371, 357, 342] W/(K*m)  temp_TLU=[200, 273, 400, 600, 800, 1000, 1200] K  T_specify=off  T_priority=None  T=0 K  T_nominal_specify=off  T_nominal_value=1  T_nominal_unit=K  Q_specify=off  Q_priority=None  Q=0 W  Q_nominal_specify=off  Q_nominal_value=1  Q_nominal_unit=W
  Window-Exterior Convection : fl_lib/Thermal/Thermal Elements/Convective Heat Transfer  thermal_type=foundation.enum.constant_variable.constant  area=area_window m^2  heat_tr_coeff=hc_window_exterior W/(K*m^2)  min_heat_tr_coeff=1e-3 W/(K*m^2)  T_specify=off  T_priority=None  T=0 K  T_nominal_specify=off  T_nominal_value=1  T_nominal_unit=K  Q_specify=off  Q_priority=None  Q=0 W  Q_nominal_specify=off  Q_nominal_value=1  Q_nominal_unit=W
  Window-Interior Conduction : fl_lib/Thermal/Thermal Elements/Conductive Heat Transfer  thermal_type=foundation.enum.ConstantVariableTabulated.Constant  wall_geometry=foundation.enum.ConductionWallGeometry.Planar  area=area_window m^2  thickness=thickness_window / 2 m  d_in=0.05 m  d_out=0.1 m  L=1 m  th_cond_min=10 W/(K*m)  th_cond=k_window W/(K*m)  th_cond_TLU=[413, 401, 392, 383, 371, 357, 342] W/(K*m)  temp_TLU=[200, 273, 400, 600, 800, 1000, 1200] K  T_specify=off  T_priority=None  T=0 K  T_nominal_specify=off  T_nominal_value=1  T_nominal_unit=K  Q_specify=off  Q_priority=None  Q=0 W  Q_nominal_specify=off  Q_nominal_value=1  Q_nominal_unit=W
  Window-Interior Convection : fl_lib/Thermal/Thermal Elements/Convective Heat Transfer  thermal_type=foundation.enum.constant_variable.constant  area=area_window m^2  heat_tr_coeff=hc_window_interior W/(K*m^2)  min_heat_tr_coeff=1e-3 W/(K*m^2)  T_specify=off  T_priority=None  T=0 K  T_nominal_specify=off  T_nominal_value=1  T_nominal_unit=K  Q_specify=off  Q_priority=None  Q=0 W  Q_nominal_specify=off  Q_nominal_value=1  Q_nominal_unit=W
  Exterior : PMIOPort  Side=Left
  Interior : PMIOPort  Port=2  Side=Right
  connections:
  Roof-Interior Convection/LConn1 -- Roof-Interior Conduction/RConn1
  Roof-Exterior Conduction/RConn1 -- Roof-Interior Conduction/LConn1 -- Roof Thermal Mass/LConn1
  Roof-Exterior Conduction/LConn1 -- Roof-Exterior Convection/RConn1
  Wall Thermal Mass/LConn1 -- Wall-Interior Conduction/LConn1 -- Wall-Exterior Conduction/RConn1
  Wall-Interior Conduction/RConn1 -- Wall-Interior Convection/LConn1
  Wall-Exterior Conduction/LConn1 -- Wall-Exterior Convection/RConn1
  Window-Interior Conduction/RConn1 -- Window-Interior Convection/LConn1
  Window-Exterior Conduction/RConn1 -- Window-Interior Conduction/LConn1 -- Window Thermal Mass/LConn1
  Window-Exterior Conduction/LConn1 -- Window-Exterior Convection/RConn1
  Inside Wall Thermal Mass/LConn1 -- Inside Wall-Interior Conduction/LConn1
  Inside Wall-Interior Convection/RConn1 -- Wall-Interior Convection/RConn1 -- Roof-Interior Convection/RConn1 -- Interior/RConn1 -- Window-Interior Convection/RConn1 -- Furniture-Interior Convection/RConn1
  Inside Wall-Interior Conduction/RConn1 -- Inside Wall-Interior Convection/LConn1
  Roof-Exterior Convection/LConn1 -- Exterior/RConn1 -- Window-Exterior Convection/LConn1 -- Wall-Exterior Convection/LConn1
  Furniture-Interior Convection/LConn1 -- Furniture Thermal Mass/LConn1

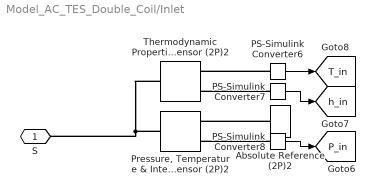
== system Model_AC_TES_Double_Coil/Inlet ==
  Absolute Reference (2P)2 : fl_lib/Two-Phase Fluid/Elements/Absolute Reference (2P)
  PS-Simulink Converter6 : nesl_utility/PS-Simulink Converter  PhysicalDomain=network_engine_domain  SubClassName=ps_output  LeftPortType=input  RightPortType=output  PseudoPeriodic=off  Frequencies=[]  VectorFormat=inherit  Unit=degC  AffineConversion=on
  PS-Simulink Converter7 : nesl_utility/PS-Simulink Converter  PhysicalDomain=network_engine_domain  SubClassName=ps_output  LeftPortType=input  RightPortType=output  PseudoPeriodic=off  Frequencies=[]  VectorFormat=inherit  Unit=inherit  AffineConversion=off
  PS-Simulink Converter8 : nesl_utility/PS-Simulink Converter  PhysicalDomain=network_engine_domain  SubClassName=ps_output  LeftPortType=input  RightPortType=output  PseudoPeriodic=off  Frequencies=[]  VectorFormat=inherit  Unit=inherit  AffineConversion=off
  "Pressure, Temperature & Internal Energy Sensor (2P)2" : fl_lib/Two-Phase Fluid/Sensors/Pressure, Temperature & Internal Energy Sensor (2P)  reference=foundation.enum.MeasurementReference.difference  pressure=true  pressure_spec=foundation.enum.PressureMeasementSpec.Absolute  temperature=false  internal_energy=false
      settings: InternalSimscapePortConfiguration="{\"Bottom\":[],\"Left\":[{\"id\":\"A\",\"label\":\"A\",\"type\":\"foundation.two_phase_fluid.two_phase_fluid\"}],\"Right\":[{\"id\":\"B\",\"label\":\"B\",\"type\":\"foundation.two_phase_fluid.two_phase_fluid\"},{\"id\":\"P\",\"label\":\"P\",\"type\":\"output\"}],\"Top\":[]}"
  Thermodynamic Properties Sensor (2P)2 : fl_lib/Two-Phase Fluid/Sensors/Thermodynamic Properties Sensor (2P)  temperature=true  enthalpy=true  density=false  specific_volume=false  entropy=false
      settings: InternalSimscapePortConfiguration="{\"Bottom\":[],\"Left\":[{\"id\":\"A\",\"label\":\"A\",\"type\":\"foundation.two_phase_fluid.two_phase_fluid\"}],\"Right\":[{\"id\":\"T\",\"label\":\"T\",\"type\":\"output\"},{\"id\":\"H\",\"label\":\"h\",\"type\":\"output\"}],\"Top\":[]}"
  S : PMIOPort  Side=Right
  tag scope: P_in=global, T_in=global, h_in=global
  wires:
  PS-Simulink Converter8/1 -> [P_in]
  PS-Simulink Converter7/1 -> [h_in]
  PS-Simulink Converter6/1 -> [T_in]
  connections:
  Thermodynamic Properties Sensor (2P)2/LConn1 -- "Pressure, Temperature & Internal Energy Sensor (2P)2"/LConn1 -- S/RConn1
  Absolute Reference (2P)2/LConn1 -- "Pressure, Temperature & Internal Energy Sensor (2P)2"/RConn1
  PS-Simulink Converter7/LConn1 -- Thermodynamic Properties Sensor (2P)2/RConn2
  PS-Simulink Converter8/LConn1 -- "Pressure, Temperature & Internal Energy Sensor (2P)2"/RConn2
  PS-Simulink Converter6/LConn1 -- Thermodynamic Properties Sensor (2P)2/RConn1

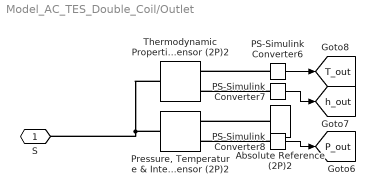
== system Model_AC_TES_Double_Coil/Outlet ==
  Absolute Reference (2P)2 : fl_lib/Two-Phase Fluid/Elements/Absolute Reference (2P)
  PS-Simulink Converter6 : nesl_utility/PS-Simulink Converter  PhysicalDomain=network_engine_domain  SubClassName=ps_output  LeftPortType=input  RightPortType=output  PseudoPeriodic=off  Frequencies=[]  VectorFormat=inherit  Unit=degC  AffineConversion=on
  PS-Simulink Converter7 : nesl_utility/PS-Simulink Converter  PhysicalDomain=network_engine_domain  SubClassName=ps_output  LeftPortType=input  RightPortType=output  PseudoPeriodic=off  Frequencies=[]  VectorFormat=inherit  Unit=inherit  AffineConversion=off
  PS-Simulink Converter8 : nesl_utility/PS-Simulink Converter  PhysicalDomain=network_engine_domain  SubClassName=ps_output  LeftPortType=input  RightPortType=output  PseudoPeriodic=off  Frequencies=[]  VectorFormat=inherit  Unit=inherit  AffineConversion=off
  "Pressure, Temperature & Internal Energy Sensor (2P)2" : fl_lib/Two-Phase Fluid/Sensors/Pressure, Temperature & Internal Energy Sensor (2P)  reference=foundation.enum.MeasurementReference.difference  pressure=true  pressure_spec=foundation.enum.PressureMeasementSpec.Absolute  temperature=false  internal_energy=false
      settings: InternalSimscapePortConfiguration="{\"Bottom\":[],\"Left\":[{\"id\":\"A\",\"label\":\"A\",\"type\":\"foundation.two_phase_fluid.two_phase_fluid\"}],\"Right\":[{\"id\":\"B\",\"label\":\"B\",\"type\":\"foundation.two_phase_fluid.two_phase_fluid\"},{\"id\":\"P\",\"label\":\"P\",\"type\":\"output\"}],\"Top\":[]}"
  Thermodynamic Properties Sensor (2P)2 : fl_lib/Two-Phase Fluid/Sensors/Thermodynamic Properties Sensor (2P)  temperature=true  enthalpy=true  density=false  specific_volume=false  entropy=false
      settings: InternalSimscapePortConfiguration="{\"Bottom\":[],\"Left\":[{\"id\":\"A\",\"label\":\"A\",\"type\":\"foundation.two_phase_fluid.two_phase_fluid\"}],\"Right\":[{\"id\":\"T\",\"label\":\"T\",\"type\":\"output\"},{\"id\":\"H\",\"label\":\"h\",\"type\":\"output\"}],\"Top\":[]}"
  S : PMIOPort  Side=Left
  tag scope: P_out=global, T_out=global, h_out=global
  wires:
  PS-Simulink Converter8/1 -> [P_out]
  PS-Simulink Converter7/1 -> [h_out]
  PS-Simulink Converter6/1 -> [T_out]
  connections:
  Thermodynamic Properties Sensor (2P)2/LConn1 -- "Pressure, Temperature & Internal Energy Sensor (2P)2"/LConn1 -- S/RConn1
  Absolute Reference (2P)2/LConn1 -- "Pressure, Temperature & Internal Energy Sensor (2P)2"/RConn1
  PS-Simulink Converter7/LConn1 -- Thermodynamic Properties Sensor (2P)2/RConn2
  PS-Simulink Converter8/LConn1 -- "Pressure, Temperature & Internal Energy Sensor (2P)2"/RConn2
  PS-Simulink Converter6/LConn1 -- Thermodynamic Properties Sensor (2P)2/RConn1

== system Model_AC_TES_Double_Coil/Q_Charge ==
  Plus : Sum  Inputs=+-
  Product : Product
  Q : Outport
  wires:
  [h_out] -> Plus/1
  [f_r32_TES] -> Product/1
  Plus/1 -> Product/2
  [h_in] -> Plus/2
  Product/1 -> Q/1

== system Model_AC_TES_Double_Coil/Q_Charge1 ==
  Plus : Sum  Inputs=+-
  Product : Product
  Q : Outport
  wires:
  [h_out] -> Plus/1
  [f_r32_TES] -> Product/1
  Plus/1 -> Product/2
  [h_in] -> Plus/2
  Product/1 -> Q/1
